simulink model "state_Harness3"  (R2023b)
settings: Solver=FixedStepAuto  StartTime=0.0  StopTime=240  FixedStep=0.5  RelTol=1e-3
settings Model: Creator=miche  LastModifiedBy=miche

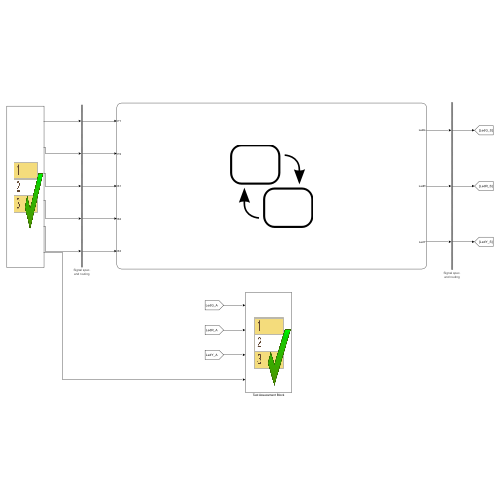
[thumbnail: Simulink's stored preview of the top-level diagram]
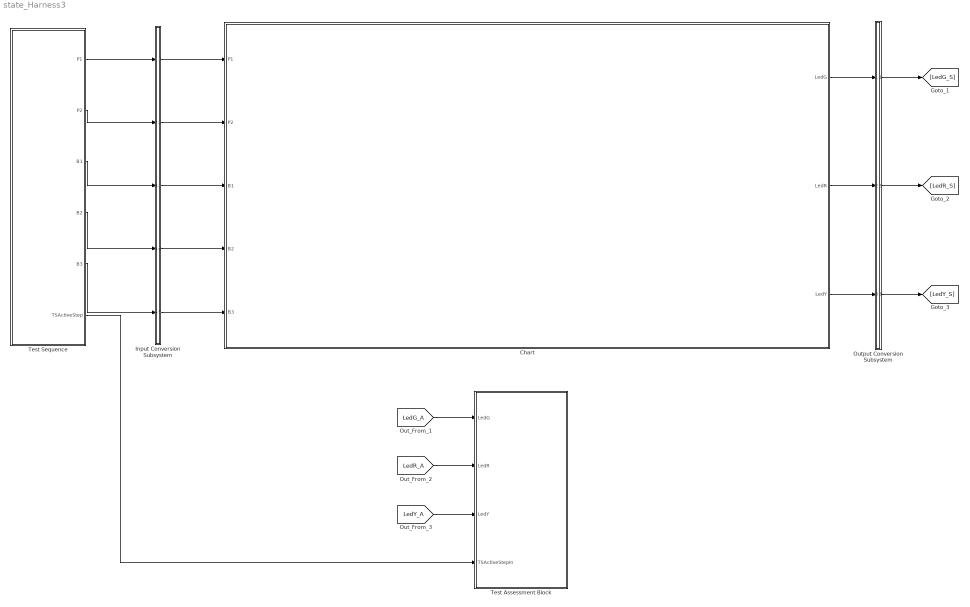
== system state_Harness3 ==
  Chart : Stateflow chart  TreatAsAtomicUnit=on
  Input Conversion Subsystem : Subsystem  Tag=__SLT_ICS__  Description=|
      | Signal spec.
      | and routing
      settings: AttributesFormatString=%<Description>
  Output Conversion Subsystem : Subsystem  Tag=__SLT_OCS__  Description=|
      | Signal spec.
      | and routing
      settings: AttributesFormatString=%<Description>
  Test Assessment Block : Test Sequence  Tag=__SLT_ASMT__  TreatAsAtomicUnit=on
  Test Sequence : Test Sequence  TreatAsAtomicUnit=on
  wires:
  [LedG_A] -> Test Assessment Block/1(LedG)
  [LedR_A] -> Test Assessment Block/2(LedR)
  [LedY_A] -> Test Assessment Block/3(LedY)
  Test Sequence/1(P1) -> Input Conversion Subsystem/1(Inport_1)
  Test Sequence/2(P2) -> Input Conversion Subsystem/2(Inport_2)
  Test Sequence/3(B1) -> Input Conversion Subsystem/3(Inport_3)
  Test Sequence/4(B2) -> Input Conversion Subsystem/4(Inport_4)
  Test Sequence/5(B3) -> Input Conversion Subsystem/5(Inport_5)
  Output Conversion Subsystem/1(Outport_1) -> [LedG_S]
  Output Conversion Subsystem/2(Outport_2) -> [LedR_S]
  Output Conversion Subsystem/3(Outport_3) -> [LedY_S]
  Input Conversion Subsystem/1(Outport_1) -> Chart/1(P1)
  Input Conversion Subsystem/2(Outport_2) -> Chart/2(P2)
  Input Conversion Subsystem/3(Outport_3) -> Chart/3(B1)
  Input Conversion Subsystem/4(Outport_4) -> Chart/4(B2)
  Input Conversion Subsystem/5(Outport_5) -> Chart/5(B3)
  Chart/1(LedG) -> Output Conversion Subsystem/1(Inport_1)
  Chart/2(LedR) -> Output Conversion Subsystem/2(Inport_2)
  Chart/3(LedY) -> Output Conversion Subsystem/3(Inport_3)
  Test Sequence/6(TSActiveStep) -> Test Assessment Block/4(TSActiveStepIn)

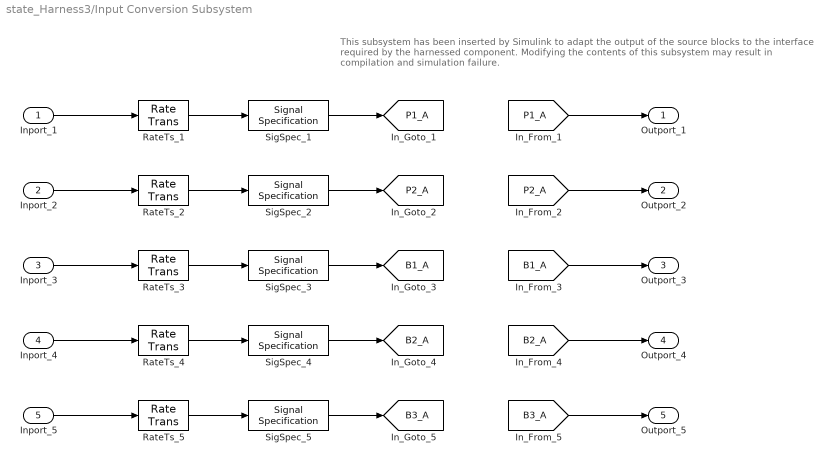
== system state_Harness3/Input Conversion Subsystem ==
  note: This subsystem has been inserted by Simulink to adapt the output of the source blocks to the interface required by the harnessed component.
      |  Modifying the contents of this subsystem may result in compilation and simulation failure.
  Inport_1 : Inport
  Inport_2 : Inport  Port=2
  Inport_3 : Inport  Port=3
  Inport_4 : Inport  Port=4
  Inport_5 : Inport  Port=5
  RateTs_{1..5} (5 alike) : RateTransition  OutPortSampleTime=[-1, 0]
  SigSpec_{1..5} (5 alike) : SignalSpecification  OutDataTypeStr=double  Dimensions=[1]  SampleTime=[-1, 0]
  Outport_1 : Outport
  Outport_2 : Outport  Port=2
  Outport_3 : Outport  Port=3
  Outport_4 : Outport  Port=4
  Outport_5 : Outport  Port=5
  tag scope: B1_A=global, B2_A=global, B3_A=global, P1_A=global, P2_A=global
  wires:
  [P1_A] -> Outport_1/1
  SigSpec_1/1 -> [P1_A]
  RateTs_1/1 -> SigSpec_1/1
  Inport_1/1 -> RateTs_1/1
  [P2_A] -> Outport_2/1
  SigSpec_2/1 -> [P2_A]
  RateTs_2/1 -> SigSpec_2/1
  Inport_2/1 -> RateTs_2/1
  [B1_A] -> Outport_3/1
  SigSpec_3/1 -> [B1_A]
  RateTs_3/1 -> SigSpec_3/1
  Inport_3/1 -> RateTs_3/1
  [B2_A] -> Outport_4/1
  SigSpec_4/1 -> [B2_A]
  RateTs_4/1 -> SigSpec_4/1
  Inport_4/1 -> RateTs_4/1
  [B3_A] -> Outport_5/1
  SigSpec_5/1 -> [B3_A]
  RateTs_5/1 -> SigSpec_5/1
  Inport_5/1 -> RateTs_5/1

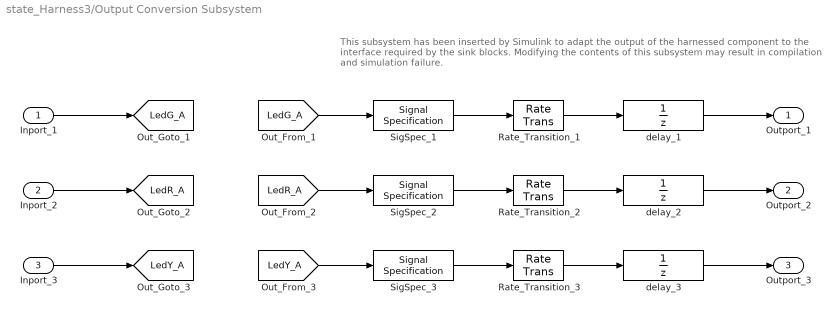
== system state_Harness3/Output Conversion Subsystem ==
  note: This subsystem has been inserted by Simulink to adapt the output of the harnessed component to the interface required by the sink blocks.
      |  Modifying the contents of this subsystem may result in compilation and simulation failure.
  Inport_1 : Inport
  Inport_2 : Inport  Port=2
  Inport_3 : Inport  Port=3
  Rate_Transition_1 : RateTransition  OutPortSampleTimeOpt=Inherit
  Rate_Transition_2 : RateTransition  OutPortSampleTimeOpt=Inherit
  Rate_Transition_3 : RateTransition  OutPortSampleTimeOpt=Inherit
  SigSpec_1 : SignalSpecification  OutDataTypeStr=double  Dimensions=[1]  SampleTime=0.5
  SigSpec_2 : SignalSpecification  OutDataTypeStr=double  Dimensions=[1]  SampleTime=0.5
  SigSpec_3 : SignalSpecification  OutDataTypeStr=double  Dimensions=[1]  SampleTime=0.5
  delay_1 : UnitDelay  SampleTime=-1
  delay_2 : UnitDelay  SampleTime=-1
  delay_3 : UnitDelay  SampleTime=-1
  Outport_1 : Outport
  Outport_2 : Outport  Port=2
  Outport_3 : Outport  Port=3
  tag scope: LedG_A=global, LedR_A=global, LedY_A=global
  wires:
  Inport_1/1 -> [LedG_A]
  [LedG_A] -> SigSpec_1/1
  SigSpec_1/1 -> Rate_Transition_1/1
  Rate_Transition_1/1 -> delay_1/1
  delay_1/1 -> Outport_1/1
  Inport_2/1 -> [LedR_A]
  [LedR_A] -> SigSpec_2/1
  SigSpec_2/1 -> Rate_Transition_2/1
  Rate_Transition_2/1 -> delay_2/1
  delay_2/1 -> Outport_2/1
  Inport_3/1 -> [LedY_A]
  [LedY_A] -> SigSpec_3/1
  SigSpec_3/1 -> Rate_Transition_3/1
  Rate_Transition_3/1 -> delay_3/1
  delay_3/1 -> Outport_3/1

== stateflow chart state_Harness3/Test Assessment Block ==
  state Run
    state VerifyInit
      verify(~LedG & ~LedR & ~LedY)
    state VerifyGateClose
      verify(~LedG & ~LedR & ~LedY)
    state VerifyGateOpening
      verify(~LedG & ~LedR & ~LedY)
    state VerifyGateOpening2
      state VerifyGateOpening2_1
        verify(~LedG & ~LedR & ~LedY)
      state VerifyGateOpening2_2
        verify(~LedG & ~LedR & LedY)
      (default) -> VerifyGateOpening2_1
      VerifyGateOpening2_1 -> VerifyGateOpening2_2 : [
          | after(2, sec)
          | ]
      VerifyGateOpening2_2 -> VerifyGateOpening2_1 : [
          | after(2, sec)
          | ]
    state VerifyGateOpen
      verify(LedG & LedR & LedY)
    state VerifyGateOpenObstacle
      verify(LedG & LedR & LedY)
    state VerifyGateOpenObstacle1
      state VerifyGateOpenObstacle1_1
        verify(~LedG & LedR & LedY)
      state VerifyGateOpenObstacle1_2
        verify(LedG & LedR & LedY)
      (default) -> VerifyGateOpenObstacle1_1
      VerifyGateOpenObstacle1_1 -> VerifyGateOpenObstacle1_2 : [
          | after(1, sec)
          | ]
      VerifyGateOpenObstacle1_2 -> VerifyGateOpenObstacle1_1 : [
          | after(1, sec)
          | ]
    state VerifyGateOpenWithoutObstacle
      verify(LedG & LedR & LedY)
    state VerifyGateClosing
      state VerifyGateClosing_1
        verify(~LedG & ~LedR & ~LedY)
      state VerifyGateClosing_2
        verify(~LedG & ~LedR & LedY)
      (default) -> VerifyGateClosing_1
      VerifyGateClosing_1 -> VerifyGateClosing_2 : [
          | after(2, sec)
          | ]
      VerifyGateClosing_2 -> VerifyGateClosing_1 : [
          | after(2, sec)
          | ]
    state VerifyGateOpenClosed
      verify(~LedG & ~LedR & ~LedY)
    state step_1_2
    (default) -> (junction 22)
    Run -> (junction 22)
    (junction 22) -> (junction 23) [order 1] : [TSActiveStepIn == TSActiveStepEnumH3.Init
        | ]
    (junction 23) -> VerifyInit [order 1] : [~in(Run.VerifyInit)]
    (junction 22) -> (junction 51) [order 2]
    (junction 23) -> (junction 26) [order 2]
    (junction 51) -> (junction 52) [order 1] : [TSActiveStepIn == TSActiveStepEnumH3.GateClose
        | ]
    (junction 52) -> VerifyGateClose [order 1] : [~in(Run.VerifyGateClose)]
    (junction 51) -> (junction 60) [order 2]
    (junction 52) -> (junction 55) [order 2]
    (junction 60) -> (junction 61) [order 1] : [TSActiveStepIn == TSActiveStepEnumH3.GateOpening
        | ]
    (junction 61) -> VerifyGateOpening [order 1] : [~in(Run.VerifyGateOpening)]
    (junction 60) -> (junction 69) [order 2]
    (junction 61) -> (junction 64) [order 2]
    (junction 69) -> (junction 70) [order 1] : [TSActiveStepIn == TSActiveStepEnumH3.GateOpening2
        | ]
    (junction 70) -> VerifyGateOpening2 [order 1] : [~in(Run.VerifyGateOpening2)]
    (junction 69) -> (junction 87) [order 2]
    (junction 70) -> (junction 73) [order 2]
    (junction 87) -> (junction 88) [order 1] : [TSActiveStepIn == TSActiveStepEnumH3.GateOpen
        | ]
    (junction 88) -> VerifyGateOpen [order 1] : [~in(Run.VerifyGateOpen)]
    (junction 87) -> (junction 96) [order 2]
    (junction 88) -> (junction 91) [order 2]
    (junction 96) -> (junction 97) [order 1] : [TSActiveStepIn == TSActiveStepEnumH3.GateOpenObstacle
        | ]
    (junction 97) -> VerifyGateOpenObstacle [order 1] : [~in(Run.VerifyGateOpenObstacle)]
    (junction 96) -> (junction 105) [order 2]
    (junction 97) -> (junction 100) [order 2]
    (junction 105) -> (junction 106) [order 1] : [TSActiveStepIn == TSActiveStepEnumH3.GateOpenObstacle1
        | ]
    (junction 106) -> VerifyGateOpenObstacle1 [order 1] : [~in(Run.VerifyGateOpenObstacle1)]
    (junction 105) -> (junction 123) [order 2]
    (junction 106) -> (junction 109) [order 2]
    (junction 123) -> (junction 124) [order 1] : [TSActiveStepIn == TSActiveStepEnumH3.GateOpenWithoutObstacle
        | ]
    (junction 124) -> VerifyGateOpenWithoutObstacle [order 1] : [~in(Run.VerifyGateOpenWithoutObstacle)]
    (junction 123) -> (junction 132) [order 2]
    (junction 124) -> (junction 127) [order 2]
    (junction 132) -> (junction 133) [order 1] : [TSActiveStepIn == TSActiveStepEnumH3.GateClosing
        | ]
    (junction 133) -> VerifyGateClosing [order 1] : [~in(Run.VerifyGateClosing)]
    (junction 160) -> (junction 31) [order 2]
    (junction 133) -> (junction 136) [order 2]
    (junction 160) -> (junction 161) [order 1] : [TSActiveStepIn == TSActiveStepEnumH3.GateClosed
        | ]
    (junction 161) -> VerifyGateOpenClosed [order 1] : [~in(Run.VerifyGateOpenClosed)]
    (junction 31) -> (junction 32)
    (junction 32) -> step_1_2 [order 1] : [~in(Run.step_1_2)]
    (junction 32) -> (junction 35) [order 2]
    (junction 161) -> (junction 164) [order 2]
    (junction 132) -> (junction 160) [order 2]
  (default) -> Run
  data: LedG input double size=[1]; LedR input double size=[1]; LedY input double size=[1]; TSActiveStepIn input

== stateflow chart state_Harness3/Chart ==
  state LOGIC
    state Cancello [parallel]
      settings: executionOrder=1
      state Inattivo
        en: LedG = OFF; LedR = OFF; LedY = OFF;
        ex: Var_Inattivo = OFF;
      state Apertura
        state In_Apertura
          ex: LedY: OFF;
          state Blink_AOff
            en: LedY = OFF;
          state Blink_AOn
            en: LedY = ON;
            ex: LedY = OFF;
          (default) -> Blink_AOff
          Blink_AOff -> Blink_AOn : [after(BlinkPeriod, sec)]
          Blink_AOn -> Blink_AOff : [after(BlinkPeriod, sec)]
        state Aperto
          en: LedG = ON; LedR = ON; LedY = ON; Var_Aperto = ON;
          ex: LedG = OFF; LedR = OFF; LedY = OFF; Var_Aperto = OFF;
        state Aperto_con_ostacolo
          en: LedG = ON; LedR = ON; LedY = ON; Var_Aperto = ON;
        (default) -> In_Apertura : {Var_Aperto = OFF;}
        In_Apertura -> Aperto : [after(TL, sec)]
        Aperto -> Aperto_con_ostacolo [order 2] : [P1 == ON]
        Aperto_con_ostacolo -> Aperto : [P1 == OFF]
      state Chiusura
        state In_Chiusura
          Var_In_Chiusura = OFF;
          state Blink_COff
            en:
            LedY = OFF;
          state Blink_COn
            en: LedY = ON;
            ex: LedY = OFF;
          (default) -> Blink_COff
          Blink_COff -> Blink_COn : [after(BlinkPeriod, sec)]
          Blink_COn -> Blink_COff : [after(BlinkPeriod, sec)]
        state Chiuso
          en: LedG = OFF; LedR = OFF;
          LedY = OFF; Var_Chiuso = ON;
          ex: Var_Chiuso = OFF;
        state Errore
          state In_Errore
            state Blink_EOff
              en:
              LedY = OFF;
            state Blink_EOn
              en: LedY = ON;
              ex: LedY = OFF;
            (default) -> Blink_EOff
            Blink_EOff -> Blink_EOn : [after(BlinkPeriod, sec)]
            Blink_EOn -> Blink_EOff : [[after(BlinkPeriod, sec)]]
          state LED_Rosso_Errore
            en: LedR =  ON;
            ex: LedR = OFF;
          In_Errore -> LED_Rosso_Errore : [after(ErrDur, sec)]
          (default) -> In_Errore
        (default) -> In_Chiusura : {Var_In_Chiusura = ON;
            | Var_Chiuso = OFF;}
        In_Chiusura -> Chiuso [order 1] : [P2 == ON && P1 == OFF]
        Errore -> Chiuso : [P2 == ON]
        In_Chiusura -> Errore [order 2] : [after(TL, sec) && P2 == OFF]
      (default) -> Inattivo : {Var_Inattivo = ON;
          | Var_Aperto = OFF;
          | Var_Chiuso = OFF;}
      Inattivo -> Chiusura : [(P1==OFF && P2 == OFF) ||  (P1 == ON && P2 == OFF) || (P1 == OFF && P2 == ON)]
      In_Chiusura -> Apertura [order 3] : [P1 == ON]
      Chiusura -> Apertura : [(buttonpressed1 && P1 == OFF)]
      Aperto -> Chiusura [order 1] : [after(TC, sec) && P1 == OFF]
      Apertura -> Chiusura : [buttonpressed1 && P1 == OFF]
    state Regolazione_Tempo_Lavoro [parallel]
      settings: executionOrder=2
      state Tempo_Lavoro
      state Aggiunta_Tempo_Lavoro
        en: TL = mod(TL, 120)+10
      (default) -> Tempo_Lavoro : {TL=10;}
      Aggiunta_Tempo_Lavoro -> Tempo_Lavoro
      Tempo_Lavoro -> Aggiunta_Tempo_Lavoro : [Var_Chiuso && buttonpressed3]
    state Regolazione_Tempo_Chiusura [parallel]
      settings: executionOrder=7
      state Tempo_Chiusura
      state Aggiunta_Tempo_Chiusura
        en: TC = mod(TC, 120)+10
      (default) -> Tempo_Chiusura : {TC = 10;}
      Aggiunta_Tempo_Chiusura -> Tempo_Chiusura
      Tempo_Chiusura -> Aggiunta_Tempo_Chiusura : [Var_Chiuso && buttonpressed2]
    state Ostacolo [parallel]
      settings: executionOrder=3
      state Fermo
      state Ostacolo_Presente
        state Blink_OOff
          en:
          LedG = OFF;
        state Blink_OOn
          en: LedG = ON;
          ex: LedG = OFF;
        (default) -> Blink_OOff
        Blink_OOff -> Blink_OOn : [after(BlinkPeriod2, sec)]
        Blink_OOn -> Blink_OOff : [[after(BlinkPeriod2, sec)]]
      state Aperto_Con_Ostacolo_Led
        en: LedG = ON;
      (default) -> Fermo
      Ostacolo_Presente -> Fermo [order 2] : [P1 == OFF || after(GreenDur, sec) && Var_Aperto == OFF]
      Fermo -> Ostacolo_Presente : [(Var_Inattivo || Var_Chiuso || Var_Aperto) && buttonpressed1 && P1 == ON]
      Aperto_Con_Ostacolo_Led -> Fermo
      Ostacolo_Presente -> Aperto_Con_Ostacolo_Led [order 1] : [Var_Aperto && (P1 == OFF || after(GreenDur, sec))]
    state BUTTON1 [parallel]
      settings: executionOrder=4
      state RELEASED1
      state PRESSED1
      state LONGPRESSED1
        send(buttonpressed1, Cancello);
        send(buttonpressed1, Ostacolo);
      (default) -> RELEASED1
      RELEASED1 -> PRESSED1 : [B1==ON]
      LONGPRESSED1 -> RELEASED1 : [B1 == OFF]
      PRESSED1 -> LONGPRESSED1 : [B1 == OFF]
    state BUTTON2 [parallel]
      settings: executionOrder=6
      state RELEASED2
      state PRESSED2
      state LONGPRESSED2
        send(buttonpressed2, Regolazione_Tempo_Chiusura);
      (default) -> RELEASED2
      RELEASED2 -> PRESSED2 : [B2==ON]
      LONGPRESSED2 -> RELEASED2 : [B2 == OFF]
      PRESSED2 -> LONGPRESSED2 : [B2 == OFF]
    state BUTTON3 [parallel]
      settings: executionOrder=5
      state RELEASED3
      state PRESSED3
      state LONGPRESSED3
        send(buttonpressed3, Regolazione_Tempo_Lavoro);
      (default) -> RELEASED3
      RELEASED3 -> PRESSED3 : [B3==ON]
      LONGPRESSED3 -> RELEASED3 : [B3 == OFF]
      PRESSED3 -> LONGPRESSED3 : [B3 == OFF]
  data: P1 input; P2 input; B1 input; B2 input; B3 input; OFF constant double =0; ON constant double =1; ErrDur constant double =10; GreenDur constant double =30; LedG output; LedR output; LedY output; BlinkPeriod constant double =2; BlinkPeriod2 constant double =1; TC local double =10; TL local double =10; Var_Inattivo local; Var_In_Chiusura local; Var_Chiuso local; Var_Aperto local
  events: buttonpressed3 local FUNCTION_CALL_EVENT; buttonpressed2 local FUNCTION_CALL_EVENT; buttonpressed1 local FUNCTION_CALL_EVENT

== stateflow chart state_Harness3/Test Sequence ==
  settings: updateMethod=DISCRETE  sampleTime=0.5
  state Init
    %% Initialize data outputs.
    P1 = 0;
    P2 = 0;
    B1 = 0;
    B2 = 0;
    B3 = 0;
    settings: description=Si parte dallo stato inattivo
  state GateClose
    P1 = 0;
    P2 = 1;
    B1 = 0;
    B2 = 0;
    B3 = 0;
    settings: description=Il cancello risulta chiuso all'avvio
  state GateOpening
    P1 = 0;
    P2 = 0;
    B1 = 1;
    B2 = 0;
    B3 = 0;
    settings: description=L'utente preme il pulsante B1 per aprire il cancello
  state GateOpening2
    P1 = 0;
    P2 = 0;
    B1 = 0;
    B2 = 0;
    B3 = 0;
    settings: description=Durante il fronte di discesa del pulsante il cancello inizia ad aprirsi e lampeggia il LED giallo
  state GateOpen
    P1 = 0;
    P2 = 0;
    B1 = 0;
    B2 = 0;
    B3 = 0;
    settings: description=Cancello aperto dopo TL secondi e tutti i LED accesi
  state GateOpenObstacle
    P1 = 1;
    P2 = 0;
    B1 = 1;
    B2 = 0;
    B3 = 0;
    settings: description=Viene rilevato un ostacolo
  state GateOpenObstacle1
    P1 = 1;
    P2 = 0;
    B1 = 0;
    B2 = 0;
    B3 = 0;
    settings: description=Se viene rilevato un ostacolo e si tenta di aprire il cancello inizia a lampeggiare il LED verde per 30 secondi
  state GateOpenWithoutObstacle
    P1 = 0;
    P2 = 0;
    B1 = 1;
    B2 = 0;
    B3 = 0;
    settings: description=Dopo 30 secondi l'ostacolo non viene più rilevato e l'utente vuole chiudere ll cancello
  state GateClosing
    P1 = 0;
    P2 = 0;
    B1 = 0;
    B2 = 0;
    B3 = 0;
    settings: description=Il cancello è in fase di chiusura e lampeggia il LED giallo
  state GateClosed
    P1 = 0;
    P2 = 1;
    B1 = 0;
    B2 = 0;
    B3 = 0;
    settings: description=Il cancello è chiuso e si spengono tutti i LED
  (default) -> Init
  Init -> GateClose : [
      | true
      | ]
  GateClose -> GateOpening : [
      | true
      | ]
  GateOpening -> GateOpening2 : [
      | true
      | ]
  GateOpening2 -> GateOpen : [
      | after(TL, sec)
      | ]
  GateOpen -> GateOpenObstacle : [
      | true
      | ]
  GateOpenObstacle -> GateOpenObstacle1 : [
      | true
      | ]
  GateOpenObstacle1 -> GateOpenWithoutObstacle : [
      | after(30, sec)
      | ]
  GateOpenWithoutObstacle -> GateClosing : [
      | true
      | ]
  GateClosing -> GateClosed : [
      | after(TL, sec)
      | ]
  data: P1 output double size=[1]; P2 output double size=[1]; B1 output double size=[1]; B2 output double size=[1]; B3 output double size=[1]; TSActiveStep output Enum: TSActiveStepEnumH3; TL constant double =10
